simulink model "statefeedback_sim"  (R2023b)
settings: Solver=VariableStepAuto  StartTime=0.0  StopTime=10.0  RelTol=1e-3
libraries: cstblocks x2
settings Model: Creator=DELL  LastModifiedBy=DELL

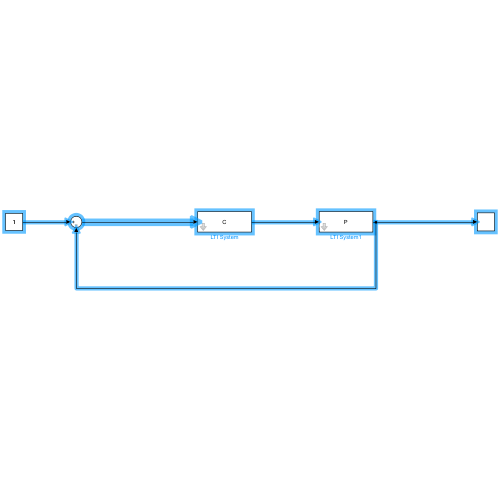
[thumbnail: Simulink's stored preview of the top-level diagram]
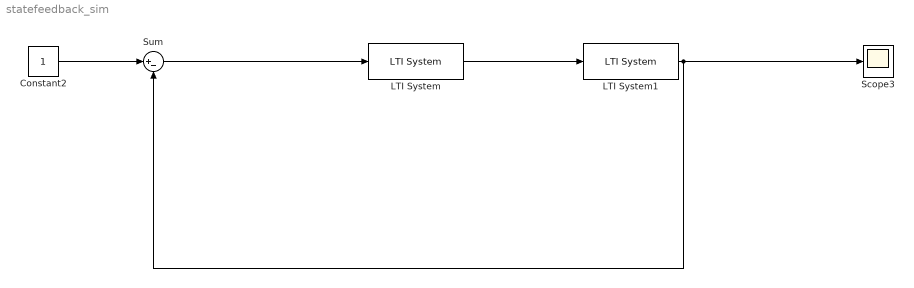
== system statefeedback_sim ==
  Constant2 : Constant
  LTI System : cstblocks/LTI System  sys=C  IC=[]  PadeOrder=0
  LTI System1 : cstblocks/LTI System  sys=P  IC=[]  PadeOrder=0
  Scope3 : Scope
  Sum : Sum  Inputs=|+-
  wires:
  Constant2/1 -> Sum/1
  LTI System/1 -> LTI System1/1
  LTI System1/1 -> Sum/2, Scope3/1
  Sum/1 -> LTI System/1
